simulink model "sampleModel2"  (R2023a)
settings: Solver=FixedStepAuto  StartTime=0.0  StopTime=10.0  RelTol=1e-3
libraries: simulink x8
settings Model: SimulationMode=software-in-the-loop (sil)  Creator=TSMC  LastModifiedBy=O
settings DataIOCC: InspectSignalLogs=on  SignalLoggingName=logsOut
settings OptimizationCC: DefaultParameterBehavior=Inlined  EnhancedBackFolding=on  PassReuseOutputArgsAs=Individual arguments  ZeroExternalMemoryAtStartup=off  ZeroInternalMemoryAtStartup=off  OptimizeBlockOrder=speed  DifferentSizesBufferReuse=on  OptimizationCustomize=off  EfficientTunableParamExpr=on
settings DebuggingCC: ParameterTunabilityLossMsg=error
settings ModelReferenceCC: UpdateModelReferenceTargets=Force
settings SFSimCC: MATLABDynamicMemAlloc=off
settings RTWCC: Description=Embedded Coder  SystemTargetFile=ert.tlc  TemplateMakefile=ert_default_tmf  GenerateReport=on  IncludeHyperlinkInReport=on  GenerateTraceInfo=on
settings CodeAppCC: ForceParamTrailComments=on  IgnoreCustomStorageClasses=off  OperatorAnnotations=on  SimulinkDataObjDesc=on  SFDataObjDesc=on  InsertBlockDesc=on
settings ERTTargetCC: TargetLangStandard=C99 (ISO)  GenerateSampleERTMain=on  SupportContinuousTime=on  InlinedParameterPlacement=NonHierarchical  ERTCustomFileTemplate=example_file_process.tlc

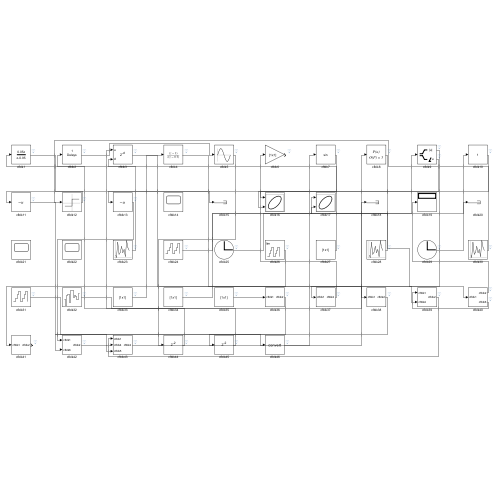
[thumbnail: Simulink's stored preview of the top-level diagram]
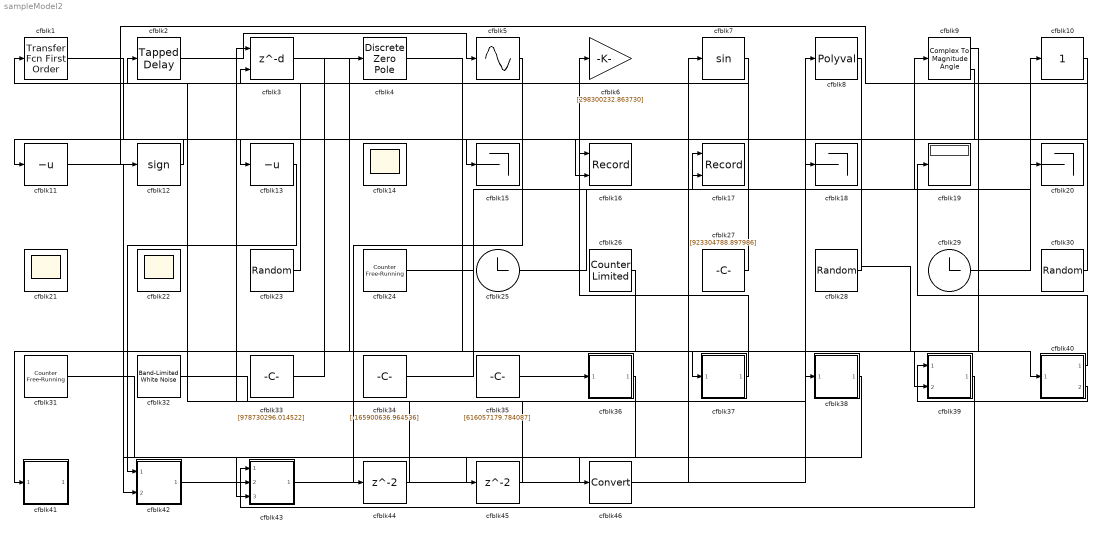
== system sampleModel2 ==
  cfblk1 : simulink/Discrete/Transfer Fcn First Order  PoleZ=0.95  ICPrevOutput=0.0  DoSatur=off
  cfblk10 : simulink/Math Operations/Slider Gain  gain=1  low=0  high=2
  cfblk11 : UnaryMinus
  cfblk12 : Signum
  cfblk13 : UnaryMinus
  cfblk14 : Scope
      settings: Floating=on
  cfblk15 : Terminator
  cfblk16 : Record  FileSettingsInternal="{\"entries\":[{\"content\":{\"excelSettings\":{\"content\":{},\"type\":\"Streamout.ExcelSettings\"}},\"type\":\"Streamout.FileSettingStorage\",\"uuid\":\"\"}],\"packageUris\":[\"http:\\/\\/schema.mathworks.com\\/mf0\\/streamout_blocks\\/R2020a\"],\"version\":\"1.0\"}"  Layout=[1 1]  SignalsInternal="{\"entries\":[{\"content\":{},\"type\":\"RecordBlkView.InputSignals\",\"uuid\":\"\"}],\"packageUris\":[\"http:\\/\\/schema.mathworks.com\\/mf0\\/streamout_blocks\\/R2020a\"],\"version\":\"1.0\"}"  VisualizationBindings="{\"xyplotplugin\":{\"info\":[{\"series\":[],\"subplotID\":1}]}}"  CompatibilityTag=XY
  cfblk17 : Record  FileSettingsInternal="{\"entries\":[{\"content\":{\"excelSettings\":{\"content\":{},\"type\":\"Streamout.ExcelSettings\"}},\"type\":\"Streamout.FileSettingStorage\",\"uuid\":\"\"}],\"packageUris\":[\"http:\\/\\/schema.mathworks.com\\/mf0\\/streamout_blocks\\/R2020a\"],\"version\":\"1.0\"}"  Layout=[1 1]  SignalsInternal="{\"entries\":[{\"content\":{},\"type\":\"RecordBlkView.InputSignals\",\"uuid\":\"\"}],\"packageUris\":[\"http:\\/\\/schema.mathworks.com\\/mf0\\/streamout_blocks\\/R2020a\"],\"version\":\"1.0\"}"  VisualizationBindings="{\"xyplotplugin\":{\"info\":[{\"series\":[],\"subplotID\":1}]}}"  CompatibilityTag=XY
  cfblk18 : Terminator
  cfblk19 : Display
  cfblk2 : simulink/Discrete/Tapped Delay  vinit=0.0  samptime=-1  NumDelays=1  DelayOrder=Oldest  includeCurrent=off
  cfblk20 : Terminator
  cfblk21 : Scope
      settings: Floating=on
  cfblk22 : Scope
      settings: Floating=on
  cfblk23 : UniformRandomNumber  Minimum=[-8899243654.253603]  Maximum=[1603305318.290040]  Seed=[19065076.000000]  SampleTime=0.1
  cfblk24 : simulink/Sources/Counter Free-Running  NumBits=[33.000000]  tsamp=-1
  cfblk25 : Clock
  cfblk26 : simulink/Sources/Counter Limited  uplimit=[161.000000]  tsamp=-1
  cfblk27 : Constant  Value=[923304788.897986]  SampleTime=1
  cfblk28 : UniformRandomNumber  Minimum=[-4179872071.000431]  Maximum=[430910711.330197]  Seed=[53663949.000000]  SampleTime=0.1
  cfblk29 : Clock
  cfblk3 : Delay  DelayLengthSource=Input port  SampleTime=1
      settings: InputPortMap=u0,p1
  cfblk30 : UniformRandomNumber  Minimum=[-4652934182.764829]  Maximum=[5802586792.278746]  Seed=[4157953.000000]  SampleTime=0.1
  cfblk31 : simulink/Sources/Counter Free-Running  NumBits=[44.000000]  tsamp=-1
  cfblk32 : simulink/Sources/Band-Limited White Noise  Cov=[3211571615.023914]  Ts=0.1  seed=[7690582387.000000]
  cfblk33 : Constant  Value=[978730296.014522]  SampleTime=1
  cfblk34 : Constant  Value=[-165900636.964536]  SampleTime=1
  cfblk35 : Constant  Value=[616057179.784087]  SampleTime=1
  cfblk36 : Subsystem
  cfblk37 : Subsystem
  cfblk38 : Subsystem
  cfblk39 : Subsystem
  cfblk4 : DiscreteZeroPole  Poles=[0 0.5]  Gain=1
  cfblk40 : Subsystem
  cfblk41 : Subsystem
  cfblk42 : Subsystem
  cfblk43 : Subsystem
  cfblk44 : Delay  SampleTime=1
  cfblk45 : Delay  SampleTime=1
  cfblk46 : DataTypeConversion  SaturateOnIntegerOverflow=off  RndMeth=Floor
  cfblk5 : Sin  TimeSource=Use external signal  SampleTime=0
  cfblk6 : Gain  Gain=[298300232.863730]
  cfblk7 : Trigonometry
  cfblk8 : Polyval  Coefs=[ +2.081618890e-019, -1.441693666e-014, +4.719686976e-010, -8.536869453e-006, +1.621573104e-001, -8.087801117e+001 ]
  cfblk9 : ComplexToMagnitudeAngle
  wires:
  cfblk33/1 -> cfblk4/1
  cfblk7/1 -> cfblk13/1
  cfblk32/1 -> cfblk8/1
  cfblk30/1 -> cfblk12/1
  cfblk12/1 -> cfblk11/1
  cfblk43/1(cfblk2) -> cfblk18/1
  cfblk29/1 -> cfblk10/1
  cfblk2/1 -> cfblk5/1
  cfblk40/1(cfblk2) -> cfblk19/1
  cfblk8/1 -> cfblk40/1(cfblk1)
  cfblk1/1 -> cfblk15/1
  cfblk28/1 -> cfblk17/1
  cfblk37/1(cfblk2) -> cfblk6/1
  cfblk39/1(cfblk2) -> cfblk43/1(cfblk1)
  cfblk35/1 -> cfblk36/1(cfblk1)
  cfblk26/1 -> cfblk41/1(cfblk1)
  cfblk27/1 -> cfblk1/1
  cfblk9/1 -> cfblk37/1(cfblk1)
  cfblk34/1 -> cfblk9/1
  cfblk24/1 -> cfblk17/2
  cfblk9/2 -> cfblk16/1
  cfblk3/1 -> cfblk38/1(cfblk1)
  cfblk25/1 -> cfblk20/1
  cfblk10/1 -> cfblk16/2
  cfblk23/1 -> cfblk3/2
  cfblk11/1 -> cfblk43/2(cfblk4)
  cfblk13/1 -> cfblk42/1(cfblk1)
  cfblk42/1(cfblk2) -> cfblk43/3(cfblk5)
  cfblk40/2(cfblk6) -> cfblk39/1(cfblk1)
  cfblk4/1 -> cfblk39/2(cfblk4)
  cfblk36/1(cfblk2) -> cfblk42/2(cfblk6)
  cfblk5/1 -> cfblk44/1
  cfblk44/1 -> cfblk2/1
  cfblk38/1(cfblk2) -> cfblk45/1
  cfblk45/1 -> cfblk3/1
  cfblk31/1 -> cfblk46/1
  cfblk46/1 -> cfblk7/1

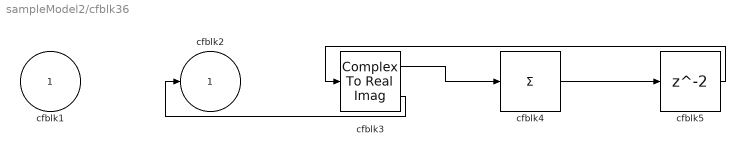
== system sampleModel2/cfblk36 ==
  cfblk1 : Inport
  cfblk3 : ComplexToRealImag
  cfblk4 : Sum  Inputs=+
  cfblk5 : Delay  SampleTime=1
  cfblk2 : Outport
  wires:
  cfblk3/1 -> cfblk4/1
  cfblk3/2 -> cfblk2/1
  cfblk4/1 -> cfblk5/1
  cfblk5/1 -> cfblk3/1

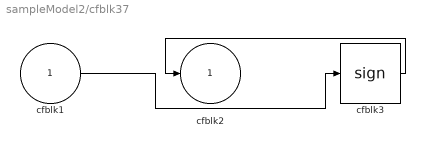
== system sampleModel2/cfblk37 ==
  cfblk1 : Inport
  cfblk3 : Signum
  cfblk2 : Outport
  wires:
  cfblk3/1 -> cfblk2/1
  cfblk1/1 -> cfblk3/1

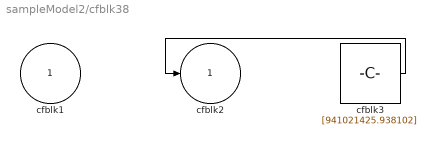
== system sampleModel2/cfblk38 ==
  cfblk1 : Inport
  cfblk3 : Constant  Value=[941021425.938102]  SampleTime=1
  cfblk2 : Outport
  wires:
  cfblk3/1 -> cfblk2/1

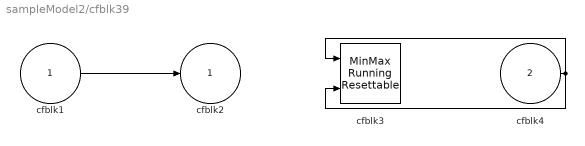
== system sampleModel2/cfblk39 ==
  cfblk1 : Inport
  cfblk4 : Inport  Port=2
  cfblk3 : simulink/Math Operations/MinMax Running Resettable  Function=min  vinit=0.0
  cfblk2 : Outport
  wires:
  cfblk1/1 -> cfblk2/1
  cfblk4/1 -> cfblk3/1, cfblk3/2

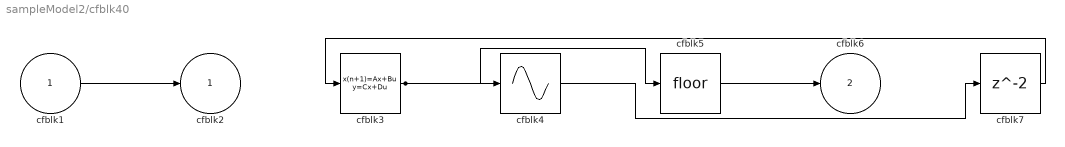
== system sampleModel2/cfblk40 ==
  cfblk1 : Inport
  cfblk3 : DiscreteStateSpace
  cfblk4 : Sin  TimeSource=Use external signal  SampleTime=0
  cfblk5 : Rounding
  cfblk7 : Delay  SampleTime=1
  cfblk2 : Outport
  cfblk6 : Outport  Port=2
  wires:
  cfblk1/1 -> cfblk2/1
  cfblk3/1 -> cfblk4/1, cfblk5/1
  cfblk5/1 -> cfblk6/1
  cfblk4/1 -> cfblk7/1
  cfblk7/1 -> cfblk3/1

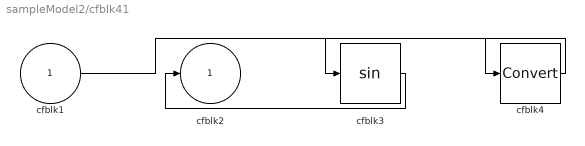
== system sampleModel2/cfblk41 ==
  cfblk1 : Inport
  cfblk3 : Trigonometry
  cfblk4 : DataTypeConversion  SaturateOnIntegerOverflow=off  RndMeth=Floor
  cfblk2 : Outport
  wires:
  cfblk3/1 -> cfblk2/1
  cfblk1/1 -> cfblk4/1
  cfblk4/1 -> cfblk3/1

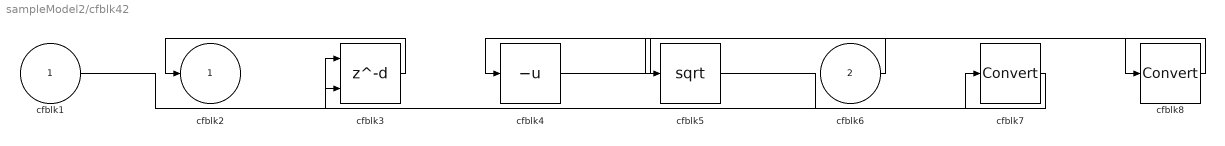
== system sampleModel2/cfblk42 ==
  cfblk1 : Inport
  cfblk6 : Inport  Port=2
  cfblk3 : Delay  DelayLengthSource=Input port  SampleTime=1
      settings: InputPortMap=u0,p1
  cfblk4 : UnaryMinus
  cfblk5 : Sqrt
  cfblk7 : DataTypeConversion  SaturateOnIntegerOverflow=off  RndMeth=Floor
  cfblk8 : DataTypeConversion  SaturateOnIntegerOverflow=off  RndMeth=Floor
  cfblk2 : Outport
  wires:
  cfblk3/1 -> cfblk2/1
  cfblk6/1 -> cfblk4/1
  cfblk1/1 -> cfblk3/1
  cfblk5/1 -> cfblk7/1
  cfblk7/1 -> cfblk3/2
  cfblk4/1 -> cfblk8/1
  cfblk8/1 -> cfblk5/1

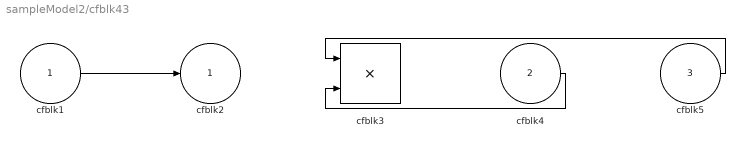
== system sampleModel2/cfblk43 ==
  cfblk1 : Inport
  cfblk4 : Inport  Port=2
  cfblk5 : Inport  Port=3
  cfblk3 : Product  Inputs=**
  cfblk2 : Outport
  wires:
  cfblk5/1 -> cfblk3/1
  cfblk1/1 -> cfblk2/1
  cfblk4/1 -> cfblk3/2
